simulink model "tank_actuator"  (R2024a)
settings: Solver=VariableStepAuto  StartTime=0.0  StopTime=20  RelTol=1e-3
values from neighbouring files (symbols this model uses):
  A = 1    [tank_actuator_init.m]
  h_0 = 4    [tank_actuator_init.m]
  K_o = 1    [tank_actuator_init.m]
  K_v = 1    [tank_actuator_init.m]
  T = 2    [tank_actuator_init.m]
settings Model: Creator=emcoates  LastModifiedBy=rune

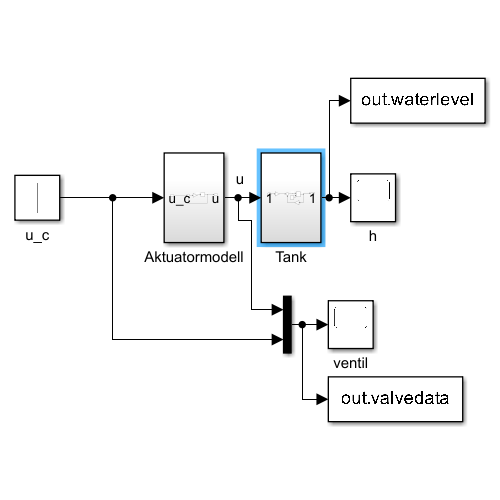
[thumbnail: Simulink's stored preview of the top-level diagram]
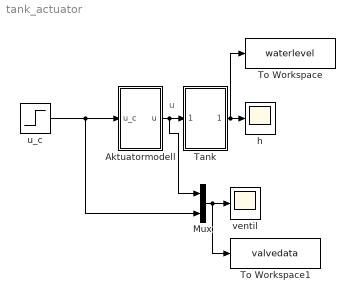
== system tank_actuator ==
  note: u
  Aktuatormodell : Subsystem
  Mux : Mux  Inputs=2
  Tank : Subsystem
  To Workspace : ToWorkspace  VariableName=waterlevel  SaveFormat=Timeseries  SampleTime=-1
  To Workspace1 : ToWorkspace  VariableName=valvedata  SaveFormat=Timeseries  SampleTime=-1
  h : Scope
  u_c : Step  SampleTime=0
  ventil : Scope
  wires:
  Tank/1(Out1) -> To Workspace/1, h/1
  Aktuatormodell/1(u) -> Mux/1, Tank/1(In1)
  Mux/1 -> To Workspace1/1, ventil/1
  u_c/1 -> Mux/2, Aktuatormodell/1(u_c)

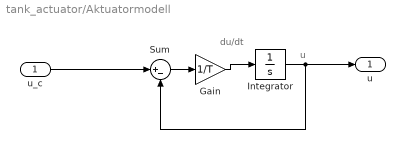
== system tank_actuator/Aktuatormodell ==
  note: du/dt
  note: u
  u_c : Inport
  Gain : Gain  Gain=1/T
  Integrator : Integrator
  Sum : Sum  Inputs=|+-
  u : Outport
  wires:
  u_c/1 -> Sum/1
  Integrator/1 -> Sum/2, u/1
  Sum/1 -> Gain/1
  Gain/1 -> Integrator/1

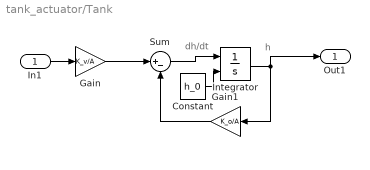
== system tank_actuator/Tank ==
  note: dh/dt
  note: h
  In1 : Inport
  Constant : Constant  Value=h_0
  Gain : Gain  Gain=K_v/A
  Gain1 : Gain  Gain=K_o/A
  Integrator : Integrator  InitialConditionSource=external  InitialCondition=h_0
  Sum : Sum  Inputs=|+-
  Out1 : Outport
  wires:
  Gain/1 -> Sum/1
  Integrator/1 -> Out1/1, Gain1/1
  Gain1/1 -> Sum/2
  In1/1 -> Gain/1
  Sum/1 -> Integrator/1
  Constant/1 -> Integrator/2
